simulink model "CascadedProblem"  (R2020b)
settings: Solver=VariableStepAuto  StartTime=0.0  StopTime=10.0  RelTol=1e-3
settings Model: Creator=baner  LastModifiedBy=baner

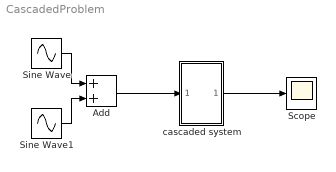
== system CascadedProblem ==
  Add : Sum
  Scope : Scope
  Sine Wave : Sin  SampleTime=0
  Sine Wave1 : Sin  Amplitude=2  Frequency=10  SampleTime=0
  cascaded system : Subsystem  TreatAsAtomicUnit=on
  wires:
  Add/1 -> cascaded system/1(In1)
  cascaded system/1(Out1) -> Scope/1
  Sine Wave/1 -> Add/1
  Sine Wave1/1 -> Add/2

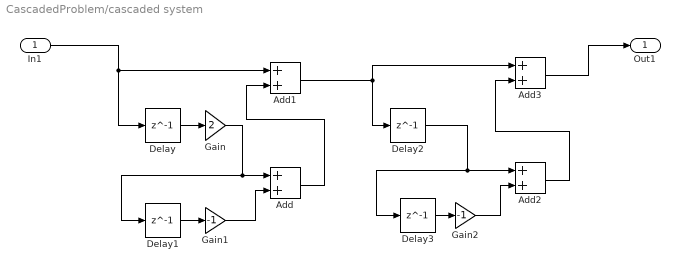
== system CascadedProblem/cascaded system ==
  In1 : Inport
  Add{,1..3} (4 alike) : Sum
  Delay{,1..3} (4 alike) : Delay  DelayLength=1
  Gain : Gain  Gain=2
  Gain1 : Gain  Gain=-1
  Gain2 : Gain  Gain=-1
  Out1 : Outport
  wires:
  Add1/1 -> Add3/1, Delay2/1
  Add/1 -> Add1/2
  Delay/1 -> Gain/1
  Gain/1 -> Delay1/1, Add/1
  Gain2/1 -> Add2/2
  Add3/1 -> Out1/1
  Delay2/1 -> Delay3/1, Add2/1
  In1/1 -> Add1/1, Delay/1
  Delay3/1 -> Gain2/1
  Add2/1 -> Add3/2
  Delay1/1 -> Gain1/1
  Gain1/1 -> Add/2
